simulink model "yaw_angle_design_step"  (R2019b)
settings: Solver=FixedStepAuto  StartTime=0.0  StopTime=step_sim_time  FixedStep=1/step_sim_freq  RelTol=1e-3
values from neighbouring files (symbols this model uses):
  disturb = 1    [rootlocus.m]
  disturb_time = 20    [rootlocus.m]
  Kp_ya = 1.2    [rootlocus.m]
  step_time = 0    [rootlocus.m]
settings Model: Creator=francois  LastModifiedBy=francois

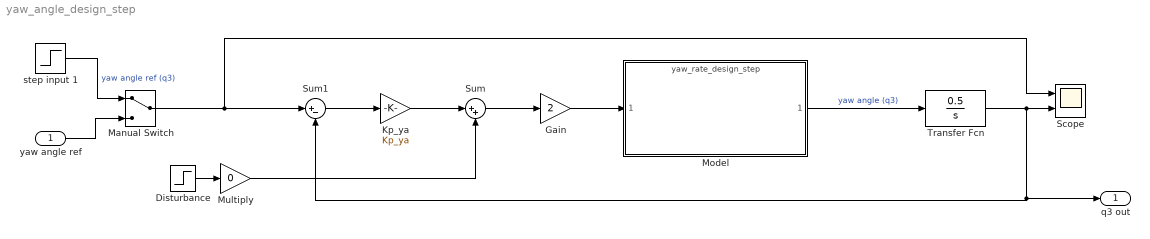
== system yaw_angle_design_step ==
  "yaw angle ref " : Inport
  "Disturbance " : Step  Time=disturb_time  After=disturb  SampleTime=0
  Gain : Gain  Gain=2
  Kp_ya : Gain  Gain=Kp_ya
  Manual Switch : ManualSwitch
  Model : ModelReference  ModelNameDialog=yaw_rate_design_step.slx  SimulationMode=Normal  ModelReferenceVersion=1.8
  Multiply : Gain  Gain=0
  Scope : Scope  NumInputPorts=2
  Sum : Sum  Inputs=|++
  Sum1 : Sum  Inputs=|+-
  Transfer Fcn : TransferFcn  Numerator=[0.5]  Denominator=[1 0]
  step input 1 : Step  Time=step_time  SampleTime=0
  "q3 out " : Outport
  wires:
  Model/1 -> Transfer Fcn/1  "yaw angle (q3)"
  Gain/1 -> Model/1
  Sum/1 -> Gain/1
  "Disturbance "/1 -> Multiply/1
  Multiply/1 -> Sum/2
  Kp_ya/1 -> Sum/1
  Sum1/1 -> Kp_ya/1
  Transfer Fcn/1 -> Sum1/2, "q3 out "/1, Scope/2
  step input 1/1 -> Manual Switch/1  "yaw angle ref (q3)"
  Manual Switch/1 -> Scope/1, Sum1/1
  "yaw angle ref "/1 -> Manual Switch/2
